simulink model "iso_calc_temp_ver2"  (R2020a)
settings: Solver=VariableStepAuto  StartTime=0.0  StopTime=inf  RelTol=1e-6
undefined symbols (not defined in the file): C, t_current, Tr, Ts, Vs, x, y, z, Zd, Zr
libraries: ros2lib x6, simulink x1
settings Model: Creator=laiy  LastModifiedBy=laiy

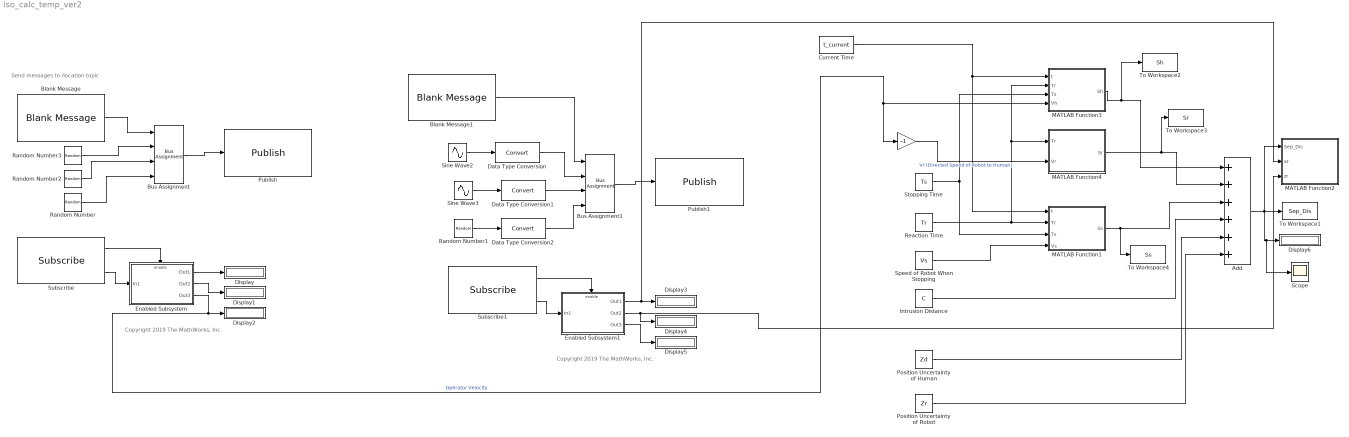
== system iso_calc_temp_ver2 ==
  note: Send messages to /location topic
  note: Copyright 2019 The MathWorks, Inc.
  note: Copyright 2019 The MathWorks, Inc.
  " " : Gain  Gain=-1
  Add : Sum  Inputs=++++++
  Blank Message : ros2lib/Blank Message  messageType=geometry_msgs/Point  SampleTime=0.01
      settings: SourceProductBaseCode=RR
  Blank Message1 : ros2lib/Blank Message  messageType=geometry_msgs/Point32  SampleTime=0.01
      settings: SourceProductBaseCode=RR
  Bus Assignment : BusAssignment  AssignedSignals=x,y,z
  Bus Assignment1 : BusAssignment  AssignedSignals=x,y,z
  Current Time : Constant  Value=t_current
  Data Type Conversion : DataTypeConversion
  Data Type Conversion1 : DataTypeConversion
  Data Type Conversion2 : DataTypeConversion
  Display{,1..6} (7 alike) : Display
  Enabled Subsystem : Subsystem
  Enabled Subsystem1 : Subsystem
  Intrusion Distance : Constant  Value=C
  MATLAB Function1 : MATLAB Function  TreatAsAtomicUnit=on
  MATLAB Function2 : MATLAB Function  TreatAsAtomicUnit=on
  MATLAB Function3 : MATLAB Function  TreatAsAtomicUnit=on
  MATLAB Function4 : MATLAB Function  TreatAsAtomicUnit=on
  Position Uncertainty of Human : Constant  Value=Zd
  Position Uncertainty of Robot : Constant  Value=Zr
  Publish : ros2lib/Publish  topicSource=Specify your own  topic=/velocity  messageType=geometry_msgs/Point  QOSHistory=Keep last  QOSDepth=1  QOSReliability=Reliable  QOSDurability=Volatile
      settings: SourceProductBaseCode=RR
  Publish1 : ros2lib/Publish  topicSource=Specify your own  topic=/bounding_box  messageType=geometry_msgs/Point32  QOSHistory=Keep last  QOSDepth=1  QOSReliability=Reliable  QOSDurability=Volatile
      settings: SourceProductBaseCode=RR
  Random Number{,1..3} (4 alike) : RandomNumber  SampleTime=0.01
  Reaction Time : Constant  Value=Tr
  Scope : Scope
  Sine Wave2 : Sin  Phase=-pi/2  SampleTime=0.01  VectorParams1D=off
  Sine Wave3 : Sin  SampleTime=0.01
  Speed of Robot When Stopping : Constant  Value=Vs
  Stopping Time : Constant  Value=Ts
  Subscribe : ros2lib/Subscribe  topicSource=Specify your own  topic=/velocity  messageType=geometry_msgs/Point  sampleTime=0.01  QOSHistory=Keep last  QOSDepth=1  QOSReliability=Reliable  QOSDurability=Volatile
      settings: SourceProductBaseCode=RR
  Subscribe1 : ros2lib/Subscribe  topicSource=Specify your own  topic=/bounding_box  messageType=geometry_msgs/Point32  sampleTime=0.01  QOSHistory=Keep last  QOSDepth=1  QOSReliability=Reliable  QOSDurability=Volatile
      settings: SourceProductBaseCode=RR
  To Workspace1 : ToWorkspace  VariableName=Sep_Dis  SampleTime=-1
  To Workspace2 : ToWorkspace  VariableName=Sh  SampleTime=-1
  To Workspace3 : ToWorkspace  VariableName=Sr  SampleTime=-1
  To Workspace4 : ToWorkspace  VariableName=Ss  SampleTime=-1
  wires:
  MATLAB Function1/1(Ss) -> To Workspace4/1, Add/3
  MATLAB Function3/1(Sh) -> To Workspace2/1, Add/1
  MATLAB Function4/1(Sr) -> To Workspace3/1, Add/2
  Intrusion Distance/1 -> Add/4
  Position Uncertainty of Human/1 -> Add/5
  Position Uncertainty of Robot/1 -> Add/6
  Enabled Subsystem/3(Out3) -> Display2/1, MATLAB Function3/4(Vh), " "/1  "Operator Velocity"
  Reaction Time/1 -> MATLAB Function1/2(Tr), MATLAB Function4/1(Tr), MATLAB Function3/2(Tr)
  Stopping Time/1 -> MATLAB Function3/3(Ts), MATLAB Function1/3(Ts)
  " "/1 -> MATLAB Function4/2(Vr)  "Vr (Directed Speed of Robot to Human)"
  Current Time/1 -> MATLAB Function1/1(t), MATLAB Function3/1(t)
  Speed of Robot When Stopping/1 -> MATLAB Function1/4(Vs)
  Add/1 -> MATLAB Function2/1(Sep_Dis), Scope/1, Display6/1, To Workspace1/1
  Data Type Conversion2/1 -> Bus Assignment1/4
  Data Type Conversion/1 -> Bus Assignment1/2
  Enabled Subsystem1/1(Out1) -> MATLAB Function2/2(xr), Display3/1
  Sine Wave2/1 -> Data Type Conversion/1
  Subscribe1/1 -> Enabled Subsystem1/Enable
  Data Type Conversion1/1 -> Bus Assignment1/3
  Random Number1/1 -> Data Type Conversion2/1
  Enabled Subsystem1/3(Out3) -> Display5/1
  Enabled Subsystem1/2(Out2) -> MATLAB Function2/3(zr), Display4/1
  Subscribe/2 -> Enabled Subsystem/1(In1)
  Sine Wave3/1 -> Data Type Conversion1/1
  Subscribe1/2 -> Enabled Subsystem1/1(In1)
  Blank Message1/1 -> Bus Assignment1/1
  Random Number2/1 -> Bus Assignment/3
  Bus Assignment/1 -> Publish/1
  Random Number/1 -> Bus Assignment/4
  Subscribe/1 -> Enabled Subsystem/Enable
  Enabled Subsystem/1(Out1) -> Display/1
  Random Number3/1 -> Bus Assignment/2
  Enabled Subsystem/2(Out2) -> Display1/1
  Blank Message/1 -> Bus Assignment/1
  Bus Assignment1/1 -> Publish1/1

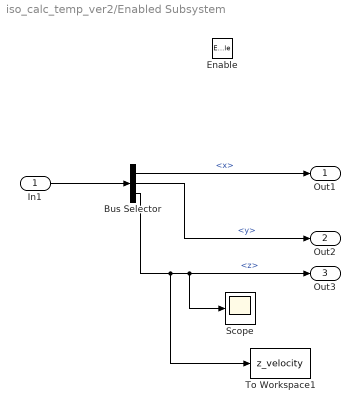
== system iso_calc_temp_ver2/Enabled Subsystem ==
  In1 : Inport
  Enable : EnablePort
  Bus Selector : BusSelector  DialogController=Simulink.DDGSource_BusSelector  OutputSignals=x,y,z
  Scope : Scope
  To Workspace1 : ToWorkspace  VariableName=z_velocity  SampleTime=-1
  Out1 : Outport  VectorParamsAs1DForOutWhenUnconnected=off
  Out2 : Outport  Port=2  VectorParamsAs1DForOutWhenUnconnected=off
  Out3 : Outport  Port=3  VectorParamsAs1DForOutWhenUnconnected=off
  wires:
  In1/1 -> Bus Selector/1
  Bus Selector/2 -> Out2/1  "<y>"
  Bus Selector/1 -> Out1/1  "<x>"
  Bus Selector/3 -> To Workspace1/1, Scope/1, Out3/1  "<z>"

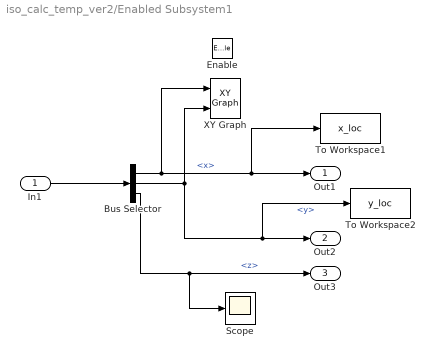
== system iso_calc_temp_ver2/Enabled Subsystem1 ==
  In1 : Inport
  Enable : EnablePort
  Bus Selector : BusSelector  DialogController=Simulink.DDGSource_BusSelector  OutputSignals=x,y,z
  Scope : Scope
  To Workspace1 : ToWorkspace  VariableName=x_loc  SampleTime=-1
  To Workspace2 : ToWorkspace  VariableName=y_loc  SampleTime=-1
  XY Graph : simulink/Sinks/XY Graph  xmin=-1  xmax=1  ymin=-1  ymax=1  st=-1
  Out1 : Outport  VectorParamsAs1DForOutWhenUnconnected=off
  Out2 : Outport  Port=2  VectorParamsAs1DForOutWhenUnconnected=off
  Out3 : Outport  Port=3  VectorParamsAs1DForOutWhenUnconnected=off
  wires:
  In1/1 -> Bus Selector/1
  Bus Selector/2 -> To Workspace2/1, Out2/1, XY Graph/2  "<y>"
  Bus Selector/1 -> To Workspace1/1, Out1/1, XY Graph/1  "<x>"
  Bus Selector/3 -> Scope/1, Out3/1  "<z>"

== matlab function iso_calc_temp_ver2/MATLAB Function4 ==
  data: Tr input; Vr input; Sr output
function Sr = fcn(Tr, Vr)

% separation distance due to robot motion
% Vr is assumed to reduces the separation distance the most

Sr = Tr * Vr;

== matlab function iso_calc_temp_ver2/MATLAB Function3 ==
  data: t input; Sh output; Tr input; Ts input; Vh input
function Sh = fcn(t, Tr, Ts, Vh)

% separation distance due to operator's change in location

%% Integral
% t_int = t:0.001:t+Tr+Ts;
% v = zeros(length(t_int),1) + Vh;
% 
% Sh = trapz(t_int,v);

%% Assuming Constant
Sh = (t+Tr+Ts) * Vh;

== matlab function iso_calc_temp_ver2/MATLAB Function1 ==
  data: t input; Tr input; Ss output; Ts input; Vs input
function Ss = fcn(t, Tr, Ts, Vs)

% separation distance due to robot stopping

%% Integral 
% t_int = t+Tr:0.001:t+Tr+Ts;
% v = zeros(length(t_int),1) + Vs;
% 
% Ss = trapz(t_int,v);

%% Assuming Constant
Ss = (t+Tr+Ts)*Vs;

== matlab function iso_calc_temp_ver2/MATLAB Function2 ==
  data: Sep_Dis input; xr input; zr input
function display(Sep_Dis, xr,zr)

%% Writing local file for server to call 
fileID = fopen('output.txt','w');
fprintf(fileID,'%f\n',Sep_Dis);
fclose(fileID);

%% Printing 
fprintf(1, 'Separation Distance: %f\n', Sep_Dis(1,1));
if sqrt(xr^2 + zr^2) <= Sep_Dis
    fprintf(1,'DANGER!!!!!!!!\n');
end
